simulink model "test_robust_mpc"  (Simulink 8.1)
settings: Solver=ode45  StartTime=0.0  StopTime=10.0  RelTol=1e-3
values from neighbouring files (symbols this model uses):
  index_row = []    [grid_ss_polytope_index.m]
  STATESGRID = []    [grid_ss_polytope_index.m]
undefined symbols (not defined in the file or in its folder): add_usys_x_d, add_usys_x_z, add_usys_y_d, add_usys_z_d, sol_x_mp_rt
settings Model: Creator=Kostas  LastModifiedBy=Kostas
settings DataIOCC: SignalLoggingSaveFormat=Dataset
settings OptimizationCC: ExpressionDepthLimit=128
settings DebuggingCC: FcnCallInpInsideContextMsg=EnableAllAsError
settings GRTTargetCC: CombineOutputUpdateFcns=on  GRTInterface=off

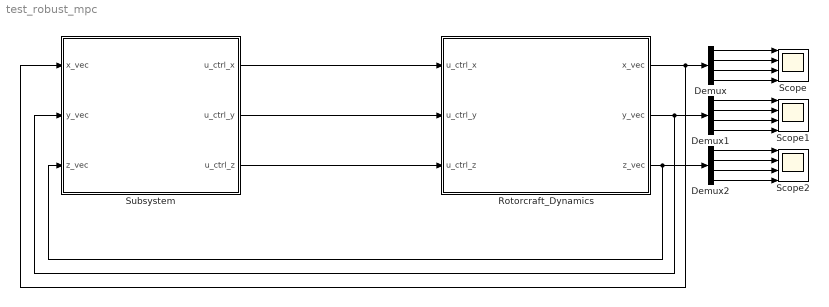
== system test_robust_mpc ==
  Demux : Demux
  Demux1 : Demux
  Demux2 : Demux
  Rotorcraft_Dynamics : Subsystem
  Scope : Scope  NumInputPorts=4
      settings: YMin=-5~-5~-5~-5  YMax=5~5~5~5
  Scope1 : Scope  NumInputPorts=4
      settings: YMin=-5~-5~-5~-5  YMax=5~5~5~5
  Scope2 : Scope  NumInputPorts=4
      settings: YMin=-5~-5~-5~-5  YMax=5~5~5~5  SaveName=ScopeData2
  Subsystem : Subsystem
  wires:
  Subsystem/1(u_ctrl_x) -> Rotorcraft_Dynamics/1(u_ctrl_x)
  Subsystem/2(u_ctrl_y) -> Rotorcraft_Dynamics/2(u_ctrl_y)
  Subsystem/3(u_ctrl_z) -> Rotorcraft_Dynamics/3(u_ctrl_z)
  Demux/1 -> Scope/1
  Demux/2 -> Scope/2
  Demux/3 -> Scope/3
  Demux/4 -> Scope/4
  Demux1/1 -> Scope1/1
  Demux1/2 -> Scope1/2
  Demux1/3 -> Scope1/3
  Demux1/4 -> Scope1/4
  Demux2/1 -> Scope2/1
  Demux2/2 -> Scope2/2
  Demux2/3 -> Scope2/3
  Demux2/4 -> Scope2/4
  Rotorcraft_Dynamics/3(z_vec) -> Subsystem/3(z_vec), Demux2/1
  Rotorcraft_Dynamics/2(y_vec) -> Subsystem/2(y_vec), Demux1/1
  Rotorcraft_Dynamics/1(x_vec) -> Subsystem/1(x_vec), Demux/1

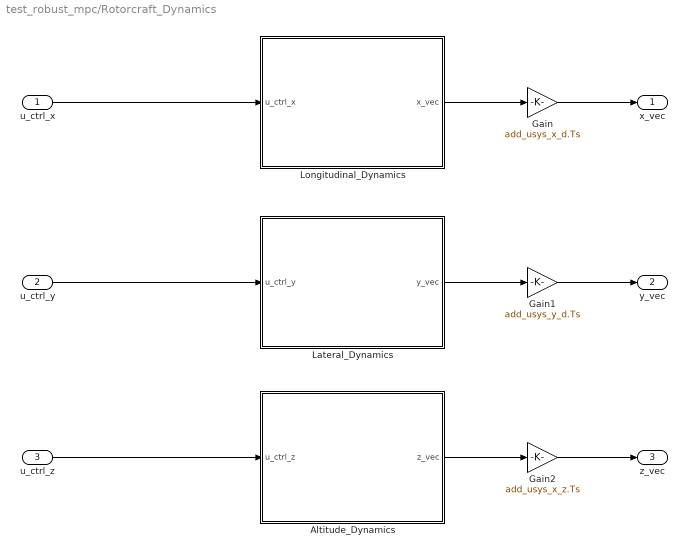
== system test_robust_mpc/Rotorcraft_Dynamics ==
  u_ctrl_x : Inport
  u_ctrl_y : Inport  Port=2
  u_ctrl_z : Inport  Port=3
  Altitude_Dynamics : Subsystem
  Gain : Gain  Gain=add_usys_x_d.Ts
  Gain1 : Gain  Gain=add_usys_y_d.Ts
  Gain2 : Gain  Gain=add_usys_x_z.Ts
  Lateral_Dynamics : Subsystem
  Longitudinal_Dynamics : Subsystem
  x_vec : Outport
  y_vec : Outport  Port=2
  z_vec : Outport  Port=3
  wires:
  Longitudinal_Dynamics/1(x_vec) -> Gain/1
  u_ctrl_x/1 -> Longitudinal_Dynamics/1(u_ctrl_x)
  u_ctrl_y/1 -> Lateral_Dynamics/1(u_ctrl_y)
  Lateral_Dynamics/1(y_vec) -> Gain1/1
  u_ctrl_z/1 -> Altitude_Dynamics/1(u_ctrl_z)
  Altitude_Dynamics/1(z_vec) -> Gain2/1
  Gain/1 -> x_vec/1
  Gain1/1 -> y_vec/1
  Gain2/1 -> z_vec/1

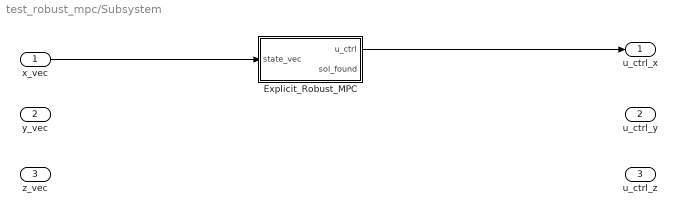
== system test_robust_mpc/Subsystem ==
  x_vec : Inport
  y_vec : Inport  Port=2
  z_vec : Inport  Port=3
  Explicit_Robust_MPC : Subsystem
  u_ctrl_x : Outport
  u_ctrl_y : Outport  Port=2
  u_ctrl_z : Outport  Port=3
  wires:
  x_vec/1 -> Explicit_Robust_MPC/1(state_vec)
  Explicit_Robust_MPC/1(u_ctrl) -> u_ctrl_x/1

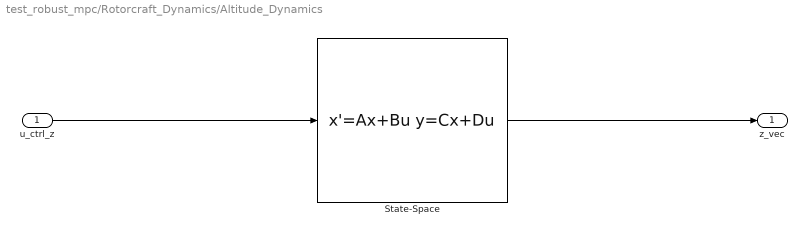
== system test_robust_mpc/Rotorcraft_Dynamics/Altitude_Dynamics ==
  u_ctrl_z : Inport
  State-Space : StateSpace  A=add_usys_z_d.continuous.matrices.A  B=add_usys_z_d.continuous.matrices.B  C=add_usys_z_d.continuous.matrices.C  D=add_usys_z_d.continuous.matrices.D  X0=zeros(length(add_usys_z_d.continuous.matrices.A),1)
  z_vec : Outport
  wires:
  u_ctrl_z/1 -> State-Space/1
  State-Space/1 -> z_vec/1

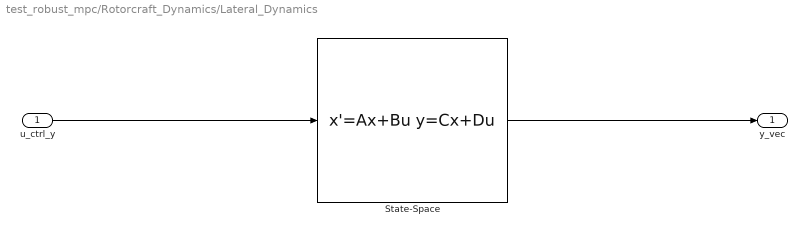
== system test_robust_mpc/Rotorcraft_Dynamics/Lateral_Dynamics ==
  u_ctrl_y : Inport
  State-Space : StateSpace  A=add_usys_y_d.continuous.matrices.A  B=add_usys_y_d.continuous.matrices.B  C=add_usys_y_d.continuous.matrices.C  D=add_usys_y_d.continuous.matrices.D  X0=zeros(length(add_usys_y_d.continuous.matrices.A),1)
  y_vec : Outport
  wires:
  u_ctrl_y/1 -> State-Space/1
  State-Space/1 -> y_vec/1

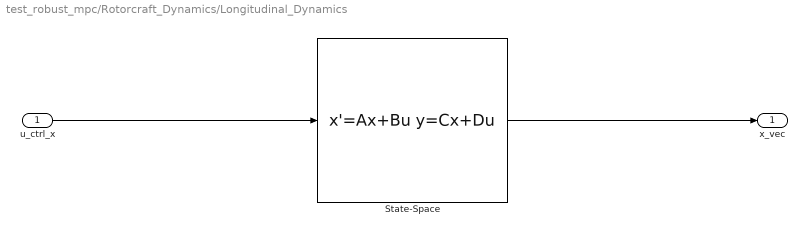
== system test_robust_mpc/Rotorcraft_Dynamics/Longitudinal_Dynamics ==
  u_ctrl_x : Inport
  State-Space : StateSpace  A=add_usys_x_d.continuous.matrices.A  B=add_usys_x_d.continuous.matrices.B  C=add_usys_x_d.continuous.matrices.C  D=add_usys_x_d.continuous.matrices.D  X0=zeros(length(add_usys_x_d.continuous.matrices.A),1)
  x_vec : Outport
  wires:
  u_ctrl_x/1 -> State-Space/1
  State-Space/1 -> x_vec/1

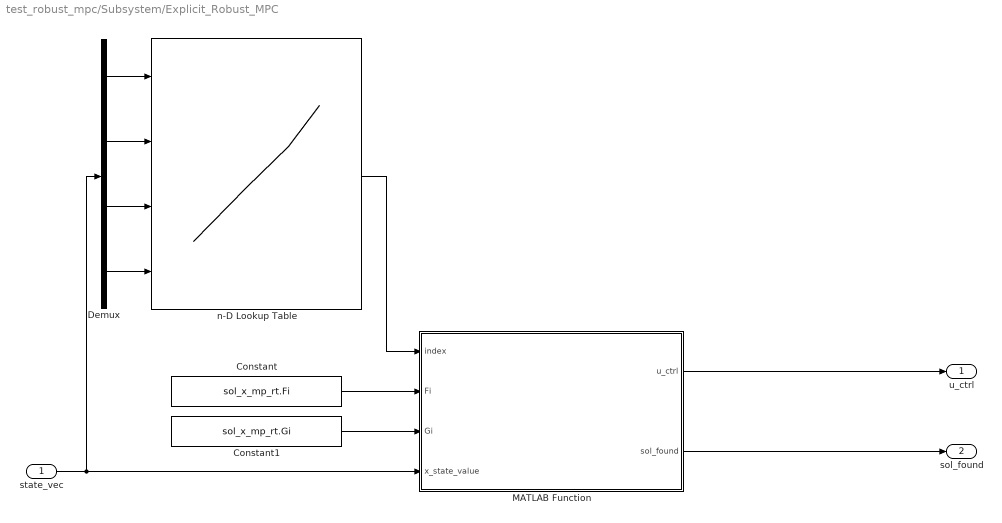
== system test_robust_mpc/Subsystem/Explicit_Robust_MPC ==
  state_vec : Inport
  Constant : Constant  Value=sol_x_mp_rt.Fi
  Constant1 : Constant  Value=sol_x_mp_rt.Gi
  Demux : Demux
  MATLAB Function : MATLAB Function  TreatAsAtomicUnit=on
  n-D Lookup Table : Lookup_n-D  NumberOfTableDimensions=4  BreakpointsForDimension1=STATESGRID.VECTORS.X1  BreakpointsForDimension2=STATESGRID.VECTORS.X2  BreakpointsForDimension3=STATESGRID.VECTORS.X3  BreakpointsForDimension4=STATESGRID.VECTORS.X4  Table=index_row  RndMeth=Simplest  InputSameDT=on
  u_ctrl : Outport
  sol_found : Outport  Port=2
  wires:
  state_vec/1 -> Demux/1, MATLAB Function/4(x_state_value)
  MATLAB Function/1(u_ctrl) -> u_ctrl/1
  MATLAB Function/2(sol_found) -> sol_found/1
  Constant/1 -> MATLAB Function/2(Fi)
  Constant1/1 -> MATLAB Function/3(Gi)
  n-D Lookup Table/1 -> MATLAB Function/1(index)
  Demux/1 -> n-D Lookup Table/1
  Demux/2 -> n-D Lookup Table/2
  Demux/3 -> n-D Lookup Table/3
  Demux/4 -> n-D Lookup Table/4

== matlab function Subsystem/Explicit_Robust_MPC/MATLAB Function ==
  data: index input double; Fi input double; Gi input double; u_ctrl output double; x_state_value input double; sol_found output double
function [u_ctrl,sol_found] = robustmpc_getInput_rt(index,Fi,Gi,x_state_value)
%#codegen

%
%   get control action from the explicit robust mpc computed using YALMIP
%
%   Syntax:
%   [u_ctrl,sol_found] = robustmpc_getInput_rt(sol_x_mp_rt, x_state_value)
%
%   Inputs:
%   sol_x_mp_rt     : RT Multiparametric Robust MPC explicit solution
%   x_state_value   : value of the state vector
%
%   Outputs:
%   u_ctrl          : control action
%   sol_found       : flag indicating whether a solution was found
%
%   Authors: Kostas Alexis (konstantinos.alexis@mavt.ethz.ch)

j = index;
if(isrow(x_state_value))
    x_state_value = x_state_value';
end

sol_found = 1;
%[i,j] = isinside(Pn, x_state_value);
if(isempty(j)==0)
    u_ctrl = Fi(j,:)*x_state_value + Gi(j,:);
    sol_found = 1;
else
    sol_found = 0;
    u_ctrl =0;
end

end
